simulink library "commrflib2"  (Simulink 6.0)
settings: Solver=ode45  SolverMode=SingleTasking  StartTime=0.0  StopTime=10.0  RelTol=1e-3
undefined symbols (not defined in the file or in its folder): Rows
libraries: dspsigattribs x12, dspmathops x2, commchan2 x2, dsparch3 x1, dspsrcs4 x1
settings Model: Creator=mikem  LastModifiedBy=mikem  ProdHWDeviceType=Microprocessor  TargetHWChar=2  TargetHWWordLengths=8,16,32,32
settings DataIOCC: SignalLoggingName=logsOut
settings OptimizationCC: BooleanDataType=off  MultiInstanced=off
settings FormatCC: IgnoreBidirectionalLines=off
settings HardwareCC: ProdHWDeviceType=Microprocessor  ShiftRightIntArith=on  TargetHWCharacteristics=InheritFromRTWHook
settings CodeAppCC: FileBanners=off
settings GRTTargetCC: TargetFcnLib=iso_c_tmw.mat  IsERTTarget=off

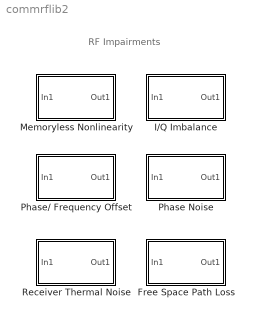
== system commrflib2 ==
  note: RF Impairments
  Free Space Path Loss : Subsystem  mask(Free Space Path Loss){mode=Distance and Frequency, dB=10, d=0.100, fc=1920}
      mask prompts: dB "Loss (dB):"; d "Distance (km):"; fc "Carrier frequency (MHz):"
      mask help:
      | Reduce the amplitude of the input signal by the amount specified.  The loss can be specified directly using the "Decibels" mode, or indirectly using the "Distance and Frequency" mode.
      |
      | The reciprocal of the loss is applied as a gain, e.g., a loss of +20 dB, which reduces the signal by a factor of 10, corresponds to a gain value of 0.1.
      |
      | Note:  The decibel amount shown on the mask is rounded for display purposes only.
      mask init:
      | if mode == 1
      | 
      | 	loss = 10.^(0.05*dB);
      | 
      | else
      | 
      | 	c = 299792458;
      | 
      | 	loss = 4*pi*d*1e3*fc*1e6/c;
      | 
      | end
      | 
      | g = 1/loss;
      | 
      | lossdB = 20*log10(loss);
      | 
      | 
      | 
      | if isempty(dB) | (sum(size(dB)) > 2),
      | 
      | 	dB = 0; g = 0;
      | 
      | 	s = ['Free Space\nPath Loss'];
      | 
      | else
      | 
      | 	s = sprintf('Free Space\nPath Loss\n%0.0f dB',lossdB);
      | 
      | end
      mask Help: helpview(commbhelp)
      mask StyleString: popup(Decibels|Distance and Frequency),edit,edit,edit
      mask CallbackString:
      | if strcmp(get_param(gcb,'mode'),'Decibels'),
      | 
      | 	set_param(gcb,'maskvisibilities',{'on' 'on' 'off' 'off'});
      | 
      | else
      | 
      | 	set_param(gcb,'maskvisibilities',{'on' 'off' 'on' 'on'});
      | 
      | end|||
      mask Display: fprintf(s)
  I/Q Imbalance : Subsystem  mask(I/Q Imbalance){ampImbal=0, phsImbal=0, Idc=0, Qdc=0}
      mask prompts: ampImbal "I/Q amplitude imbalance (dB):"; phsImbal "I/Q phase imbalance (deg):"; Idc "I dc offset:"; Qdc "Q dc offset:"
      mask help: Complex baseband model of the signal impairments caused by imbalances between in-phase and quadrature receiver components.
      mask init:
      | Igain = 10.^(0.5*[ampImbal]*.05);
      | Qgain = 10.^(0.5*[-ampImbal]*.05);
      mask Help: helpview(commbhelp)
      mask Display: disp('I/Q\nImbalance');
  Memoryless Nonlinearity : Subsystem  mask(Memoryless Nonlinearity){model_select=Cubic polynomial, linGaindB=0, GindB=0, iip3=30, am2pm=0, amam=[2.1587 1.1517], ampm=[4.0033 9.1040], x=[8.1081 1.5413 6.5202 -0.0718], y=[4.6645 2.0965 10.88 -0.003], p=0.5, GoutdB=0, vsat=1}
      mask prompts: model_select "Method:"; linGaindB "Linear gain (dB):"; GindB "Input scaling (dB):"; iip3 "IIP3 (dBm):"; am2pm "AM/PM conversion (degrees per dB):"; amam "AM/AM parameters [alpha beta]:"; ampm "AM/PM parameters [alpha beta]:"; x "AM/AM parameters [x1 x2 x3 x4]:"; y "AM/PM parameters [y1 y2 y3 y4]:"; p "Smoothness factor:"; GoutdB "Output scaling (dB):"; vsat "Output saturation level:"
      mask help:
      | Complex baseband model of memoryless nonlinearity.
      |
      | Two of the five methods (Cubic Polynomial and Hyperbolic Tangent) fit curves to measured data provided by the gain and third order intercept point (IIP3) parameters.
      |
      | The other three methods use models originated by Saleh, Ghorbani, and Rapp.  The Saleh and Ghorbani models are based on normalized nonlinear transfer functions.  Use the Input scaling and Output scaling parameters to adjust signal levels up or down from their normalized values.
      mask init:
      | switch model_select
      | case 'Cubic polynomial'
      |     str = ['Cubic\nPolynomial'];
      |     method = 1;
      | 	c1 = 10^(linGaindB/20);
      |     inputGain = sqrt(3/(10^((iip3-30)/10)));
      |     outputGain = c1/inputGain;
      | case 'Hyperbolic tangent'
      |     str = ['Hyperbolic\nTangent'];
      |     method = 2;
      | 	c1 = 10^(linGaindB/20);
      |     inputGain = sqrt(3/(10^((iip3-30)/10)));
      |     outputGain = c1/inputGain;
      | case 'Saleh model',
      |     str = ['Saleh\nModel'];
      |     method = 3;
      |     inputGain = 10^(GindB/20);
      |     outputGain = 10^(GoutdB/20);
      | case 'Ghorbani model',
      |     str = ['Ghorbani\nModel'];
      |     method = 4;
      |     inputGain = 10^(GindB/20);
      |     outputGain = 10^(GoutdB/20);
      | case 'Rapp model',
      |     str = ['Rapp\nModel'];
      |     method = 5;
      | 	c1 = 10^(linGaindB/20);
      |     inputGain = c1;
      |     outputGain = 1;
      | end
      mask Help: helpview(commbhelp)
      mask StyleString: popup(Cubic polynomial|Hyperbolic tangent|Saleh model|Ghorbani model|Rapp model),edit,edit,edit,edit,edit,edit,edit,edit,edit,edit,edit
      mask CallbackString:
      | model_type = get_param(gcb,'model_select');
      | 
      | switch model_type
      | 
      | case 'Cubic polynomial',
      | 
      | 	set_param(gcb,'maskvisibilities',{'on' 'on' 'off' 'on' 'on' 'off' 'off' 'off' 'off' 'off' 'off' 'off'});
      | 
      | case 'Hyperbolic tangent',
      | 
      | 	set_param(gcb,'maskvisibilities',{'on' 'on' 'off' 'on' 'on' 'off' 'off' 'off' 'off' 'off' 'off' 'off'});
      | 
      | case 'Saleh model',
      | 
      | 	set_param(gcb,'maskvisibilities',{'on' 'off' 'on' 'off' 'off' 'on' 'on' 'off' 'off' 'off' 'on' 'off'});
      | 
      | case 'Ghorbani model',
      | 
      | 	set_param(gcb,'maskvisibilities',{'on' 'off' 'on' 'off' 'off' 'off' 'off' 'on' 'on' 'off' 'on' 'off'});
      | 
      | case 'Rapp model',
      | 
      | 	set_param(gcb,'maskvisibilities',{'on' 'on' 'off' 'off' 'off' 'off' 'off' 'off' 'off' 'on' 'off' 'on'});
      | 
      | end|||||||||||
      mask Display: disp(str);
  Phase Noise : Subsystem  mask(Phase Noise){PhNs=-120, Fo=100, seed=2137}
      mask prompts: PhNs "Phase noise level (dBc/Hz):"; Fo "Frequency offset (Hz):"; seed "Initial seed:"
      mask help:
      | Complex baseband model of receiver phase noise.
      |
      | The output of this block is noise with a spectrum characterized by a 1/f slope.  The level of the spectrum is specified by the noise power contained in a one hertz bandwidth offset from the carrier by a certain frequency.
      mask init:
      | if PhNs>0,
      | 	error('Phase noise level should be negative.');
      | end
      | num = sqrt(2*pi*Fo*10^((PhNs)/10));
      | if num>.1,
      | 	warning('Current parameters in phase noise block may produce inaccurate results.');
      | end
      | num_taps = 64;
      | den = zeros(1,num_taps);
      | den(1) = 1;
      | for idx = 2:num_taps
      |    den(idx) = (idx - 2.5) * den(idx-1) / (idx-1);
      | end
      settings: AttributesFormatString=\n
      mask Help: helpview(commbhelp)
      mask Display: disp('Phase\nNoise');
  Phase/ Frequency Offset : Subsystem  mask(Phase/Frequency Offset){freqOffset=0, phaseOffset=0}
      mask prompts: freqOffset "Frequency offset (Hz):"; phaseOffset "Phase offset (deg):"
      mask help: Complex baseband model of residual phase and frequency offsets.
      mask Help: helpview(commbhelp)
      mask Display: disp('Phase/\nFrequency\nOffset');
  Receiver Thermal Noise : Subsystem  mask(Receiver Thermal Noise){method=Noise temperature, ntemp=290, nfigure=3.01, nfactor=2, seed=67987}
      mask prompts: method "Specification method:"; ntemp "Noise temperature (K):"; nfigure "Noise figure (dB):"; nfactor "Noise factor:"; seed "Initial seed:"
      mask help:
      | Complex baseband model of receiver thermal noise.
      |
      | The amount of noise added to the input signal may be specified either in terms of noise temperature, noise figure, or noise factor.
      mask init:
      | k=1.380650e-23; % Boltzmann's constant, J/K
      | 
      | switch method
      | case 'Noise temperature',
      | 	T = ntemp;
      | 	str = ['Noise\nTemperature\n' num2str(ntemp) ' K'];
      | case 'Noise figure',
      | 	nfactor = 10.^(0.1*nfigure);
      | 	T = 290*(nfactor-1);
      | 	str = ['Noise\nFigure\n' num2str(nfigure) ' dB'];
      | case 'Noise factor',
      | 	T = 290*(nfactor-1);
      | 	str = ['Noise\nFactor\n' num2str(nfactor)];
      | end
      | 
      | kT=k*T;
      mask Help: helpview(commbhelp)
      mask StyleString: popup(Noise temperature|Noise figure|Noise factor),edit,edit,edit,edit
      mask CallbackString:
      | method = get_param(gcb,'method');
      | 
      | switch method
      | 
      | case 'Noise temperature',
      | 
      | 	set_param(gcb,'maskvisibilities',{'on' 'on' 'off' 'off' 'on'});
      | 
      | case 'Noise figure',
      | 
      | 	set_param(gcb,'maskvisibilities',{'on' 'off' 'on' 'off' 'on'});
      | 
      | case 'Noise factor',
      | 
      | 	set_param(gcb,'maskvisibilities',{'on' 'off' 'off' 'on' 'on'});
      | 
      | end||||
      mask Display: disp(str);

== system commrflib2/Free Space Path Loss ==
  In1 : Inport
  Check Input Signal : Subsystem
      mask Display: disp('Check\nInput Signal');
  Gain : Gain  Gain=g  SaturateOnIntegerOverflow=on
  Out1 : Outport
  wires:
  In1/1 -> Check Input Signal/1(In1)
  Gain/1 -> Out1/1
  Check Input Signal/1(Out1) -> Gain/1

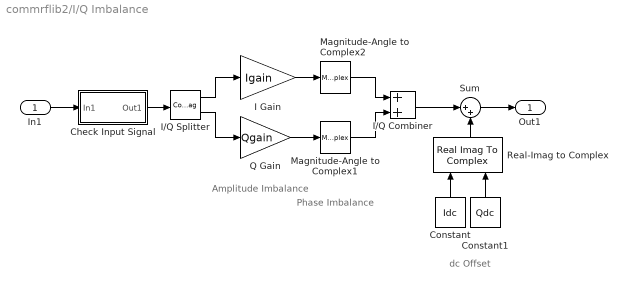
== system commrflib2/I/Q Imbalance ==
  note: Amplitude
      | Imbalance
  note: Phase
      | Imbalance
  note: dc
      | Offset
  In1 : Inport
  Check Input Signal : Subsystem
      mask Display: disp('Check\nInput Signal');
  Constant : Constant  Orientation=up  Value=Idc
  Constant1 : Constant  Orientation=up  Value=Qdc
  I Gain : Gain  Gain=Igain  SaturateOnIntegerOverflow=on
  I/Q Combiner : Sum  SaturateOnIntegerOverflow=on  InputSameDT=on
  I/Q Splitter : ComplexToRealImag
  Magnitude-Angle to Complex1 : MagnitudeAngleToComplex  Input=Magnitude  ConstantPart=pi/2+0.5*phsImbal*pi/180
  Magnitude-Angle to Complex2 : MagnitudeAngleToComplex  Input=Magnitude  ConstantPart=-0.5*phsImbal*pi/180
  Q Gain : Gain  Gain=Qgain  SaturateOnIntegerOverflow=on
  Real-Imag to Complex : RealImagToComplex  Orientation=up
  Sum : Sum  Inputs=|++  SaturateOnIntegerOverflow=on  InputSameDT=on
  Out1 : Outport
  wires:
  I/Q Splitter/1 -> I Gain/1
  I/Q Splitter/2 -> Q Gain/1
  I Gain/1 -> Magnitude-Angle to Complex2/1
  Q Gain/1 -> Magnitude-Angle to Complex1/1
  In1/1 -> Check Input Signal/1(In1)
  Sum/1 -> Out1/1
  Check Input Signal/1(Out1) -> I/Q Splitter/1
  Magnitude-Angle to Complex2/1 -> I/Q Combiner/1
  Magnitude-Angle to Complex1/1 -> I/Q Combiner/2
  I/Q Combiner/1 -> Sum/1
  Constant/1 -> Real-Imag to Complex/1
  Constant1/1 -> Real-Imag to Complex/2
  Real-Imag to Complex/1 -> Sum/2

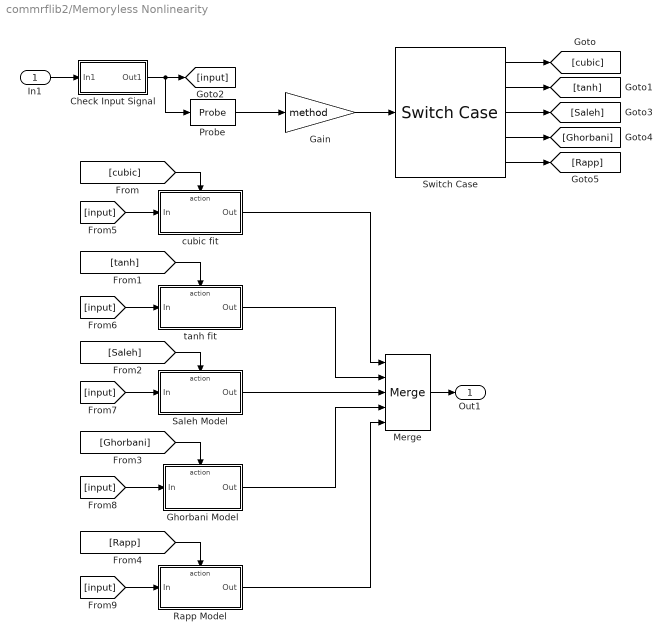
== system commrflib2/Memoryless Nonlinearity ==
  In1 : Inport
  Check Input Signal : Subsystem
      mask Display: disp('Check\nInput Signal');
  Gain : Gain  Gain=method  SaturateOnIntegerOverflow=on
  Ghorbani Model : Subsystem  TreatAsAtomicUnit=on
  Merge : Merge  Inputs=5
  Probe : Probe  ProbeWidth=off  ProbeSampleTime=off
  Rapp Model : Subsystem  TreatAsAtomicUnit=on
  Saleh Model : Subsystem  TreatAsAtomicUnit=on
  Switch Case : SwitchCase  CaseConditions={1 2 3 4 5}  CaseShowDefault=off
  cubic fit : Subsystem  TreatAsAtomicUnit=on
  tanh fit : Subsystem  TreatAsAtomicUnit=on
  Out1 : Outport
  wires:
  Gain/1 -> Switch Case/1
  Merge/1 -> Out1/1
  tanh fit/1(Out) -> Merge/2
  cubic fit/1(Out) -> Merge/1
  [cubic] -> cubic fit/Action
  [tanh] -> tanh fit/Action
  Switch Case/2 -> [tanh]
  In1/1 -> Check Input Signal/1(In1)
  Check Input Signal/1(Out1) -> [input], Probe/1
  [Rapp] -> Rapp Model/Action
  [Ghorbani] -> Ghorbani Model/Action
  [Saleh] -> Saleh Model/Action
  Switch Case/3 -> [Saleh]
  Switch Case/4 -> [Ghorbani]
  Switch Case/5 -> [Rapp]
  Saleh Model/1(Out) -> Merge/3
  Rapp Model/1(Out) -> Merge/5
  [input] -> cubic fit/1(In)
  [input] -> Rapp Model/1(In)
  [input] -> Ghorbani Model/1(In)
  [input] -> Saleh Model/1(In)
  [input] -> tanh fit/1(In)
  Ghorbani Model/1(Out) -> Merge/4
  Switch Case/1 -> [cubic]
  Probe/1 -> Gain/1

== system commrflib2/Phase Noise ==
  In1 : Inport
  Check Input Signal : Subsystem
      mask Display: disp('Check\nInput Signal');
  Digital Filter : dsparch3/Direct-Form II Transpose Filter  num=num  den=den  ic=0
  Magnitude-Angle to Complex : MagnitudeAngleToComplex  Input=Angle  ConstantPart=1
  Noise Source : Subsystem
      mask Display: disp('Noise Source')
  Product : Product  SaturateOnIntegerOverflow=on  InputSameDT=on
  Out1 : Outport
  wires:
  Noise Source/1(Out1) -> Digital Filter/1
  Product/1 -> Out1/1
  In1/1 -> Check Input Signal/1(In1)
  Magnitude-Angle to Complex/1 -> Product/2
  Digital Filter/1 -> Magnitude-Angle to Complex/1
  Check Input Signal/1(Out1) -> Product/1, Noise Source/1(In1)

== system commrflib2/Phase/ Frequency Offset ==
  In1 : Inport
  Check Input Signal : Subsystem
      mask Display: disp('Check\nInput Signal');
  Frequency Offset : Subsystem
      mask Display: disp('Frequency\nOffset');
  Phase Offset : Subsystem
      mask Display: disp('Phase\nOffset');
  Out1 : Outport
  wires:
  Frequency Offset/1(Out1) -> Out1/1
  In1/1 -> Check Input Signal/1(In1)
  Phase Offset/1(Out1) -> Frequency Offset/1(In1)
  Check Input Signal/1(Out1) -> Phase Offset/1(In1)

== system commrflib2/Receiver Thermal Noise ==
  In1 : Inport
  AWGN Noise Temp : commchan2/AWGN Channel  seed=seed  noiseMode=Variance from port  EbNodB=10  EsNodB=10  SNRdB=10  bitsPerSym=1  Ps=1  Tsym=1  variance=var
  Check Input Signal : Subsystem
      mask Display: disp('Check\nInput Signal');
  Gain : Gain  Gain=kT  SaturateOnIntegerOverflow=on
  Probe : Probe  ProbeComplexSignal=off
  Product : Product  Inputs=*/  SaturateOnIntegerOverflow=on  InputSameDT=on
  Selector : Selector  InputPortWidth=2
  Out1 : Outport
  wires:
  AWGN Noise Temp/1 -> Out1/1
  In1/1 -> Check Input Signal/1(In1)
  Probe/1 -> Product/1
  Product/1 -> Gain/1
  Gain/1 -> AWGN Noise Temp/2
  Probe/2 -> Selector/1
  Selector/1 -> Product/2
  Check Input Signal/1(Out1) -> AWGN Noise Temp/1, Probe/1

== system commrflib2/Free Space Path Loss/Check Input Signal ==
  In1 : Inport
  Check Signal Attributes : dspsigattribs/Check Signal Attributes  SigAttribCheckMethod=Does not match attributes exactly  Complexity=Complex  Frame=Ignore  DimsCheckMethod=Is...  Dimensions=Column vector (2-D) or scalar  DatatypeCheckMethod=Ignore  DatatypeGeneral=Boolean  DtypeFloatSpecific=Any floating-point  DtypeFixedSpecific=Any fixed-point  DtypeIntSpecific=Any integer  SampleMode=Ignore
  Check Signal Attributes1 : dspsigattribs/Check Signal Attributes  SigAttribCheckMethod=Matches attributes exactly  Complexity=Ignore  Frame=Sample-based  DimsCheckMethod=Is...  Dimensions=Vector (1-D or 2-D)  DatatypeCheckMethod=Ignore  DatatypeGeneral=Boolean  DtypeFloatSpecific=Any floating-point  DtypeFixedSpecific=Any fixed-point  DtypeIntSpecific=Any integer  SampleMode=Ignore
  Out1 : Outport
  wires:
  In1/1 -> Check Signal Attributes/1
  Check Signal Attributes1/1 -> Out1/1
  Check Signal Attributes/1 -> Check Signal Attributes1/1

== system commrflib2/I/Q Imbalance/Check Input Signal ==
  In1 : Inport
  Check Signal Attributes : dspsigattribs/Check Signal Attributes  SigAttribCheckMethod=Does not match attributes exactly  Complexity=Complex  Frame=Ignore  DimsCheckMethod=Is...  Dimensions=Column vector (2-D) or scalar  DatatypeCheckMethod=Ignore  DatatypeGeneral=Boolean  DtypeFloatSpecific=Any floating-point  DtypeFixedSpecific=Any fixed-point  DtypeIntSpecific=Any integer  SampleMode=Ignore
  Check Signal Attributes1 : dspsigattribs/Check Signal Attributes  SigAttribCheckMethod=Matches attributes exactly  Complexity=Ignore  Frame=Sample-based  DimsCheckMethod=Is...  Dimensions=Vector (1-D or 2-D)  DatatypeCheckMethod=Ignore  DatatypeGeneral=Boolean  DtypeFloatSpecific=Any floating-point  DtypeFixedSpecific=Any fixed-point  DtypeIntSpecific=Any integer  SampleMode=Ignore
  Out1 : Outport
  wires:
  Check Signal Attributes/1 -> Check Signal Attributes1/1
  Check Signal Attributes1/1 -> Out1/1
  In1/1 -> Check Signal Attributes/1

== system commrflib2/Memoryless Nonlinearity/Check Input Signal ==
  In1 : Inport
  Check Signal Attributes : dspsigattribs/Check Signal Attributes  SigAttribCheckMethod=Does not match attributes exactly  Complexity=Complex  Frame=Ignore  DimsCheckMethod=Is...  Dimensions=Column vector (2-D) or scalar  DatatypeCheckMethod=Ignore  DatatypeGeneral=Boolean  DtypeFloatSpecific=Any floating-point  DtypeFixedSpecific=Any fixed-point  DtypeIntSpecific=Any integer  SampleMode=Ignore
  Check Signal Attributes1 : dspsigattribs/Check Signal Attributes  SigAttribCheckMethod=Matches attributes exactly  Complexity=Ignore  Frame=Sample-based  DimsCheckMethod=Is...  Dimensions=Vector (1-D or 2-D)  DatatypeCheckMethod=Ignore  DatatypeGeneral=Boolean  DtypeFloatSpecific=Any floating-point  DtypeFixedSpecific=Any fixed-point  DtypeIntSpecific=Any integer  SampleMode=Ignore
  Out1 : Outport
  wires:
  In1/1 -> Check Signal Attributes/1
  Check Signal Attributes1/1 -> Out1/1
  Check Signal Attributes/1 -> Check Signal Attributes1/1

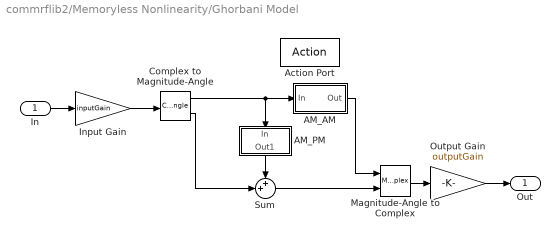
== system commrflib2/Memoryless Nonlinearity/Ghorbani Model ==
  In : Inport
  Action Port : ActionPort
  AM_AM : Subsystem
      mask Display: disp('AM/AM')
  AM_PM : Subsystem  Orientation=down
      mask Display: disp('AM/PM')
  Complex to Magnitude-Angle : ComplexToMagnitudeAngle
  Input Gain : Gain  Gain=inputGain  SaturateOnIntegerOverflow=on
  Magnitude-Angle to Complex : MagnitudeAngleToComplex
  Output Gain : Gain  Gain=outputGain  SaturateOnIntegerOverflow=on
  Sum : Sum  Inputs=++|  SaturateOnIntegerOverflow=on  InputSameDT=on
  Out : Outport
  wires:
  Sum/1 -> Magnitude-Angle to Complex/2
  AM_PM/1(Out1) -> Sum/1
  Output Gain/1 -> Out/1
  In/1 -> Input Gain/1
  Complex to Magnitude-Angle/2 -> Sum/2
  Input Gain/1 -> Complex to Magnitude-Angle/1
  Magnitude-Angle to Complex/1 -> Output Gain/1
  AM_AM/1(Out) -> Magnitude-Angle to Complex/1
  Complex to Magnitude-Angle/1 -> AM_AM/1(In), AM_PM/1(In)

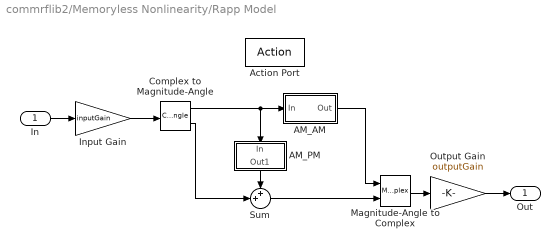
== system commrflib2/Memoryless Nonlinearity/Rapp Model ==
  In : Inport
  Action Port : ActionPort
  AM_AM : Subsystem
      mask Display: disp('AM/AM')
  AM_PM : Subsystem  Orientation=down
      mask Display: disp('AM/PM')
  Complex to Magnitude-Angle : ComplexToMagnitudeAngle
  Input Gain : Gain  Gain=inputGain  SaturateOnIntegerOverflow=on
  Magnitude-Angle to Complex : MagnitudeAngleToComplex
  Output Gain : Gain  Gain=outputGain  SaturateOnIntegerOverflow=on
  Sum : Sum  Inputs=++|  SaturateOnIntegerOverflow=on  InputSameDT=on
  Out : Outport
  wires:
  Output Gain/1 -> Out/1
  In/1 -> Input Gain/1
  Input Gain/1 -> Complex to Magnitude-Angle/1
  Magnitude-Angle to Complex/1 -> Output Gain/1
  AM_AM/1(Out) -> Magnitude-Angle to Complex/1
  Complex to Magnitude-Angle/1 -> AM_AM/1(In), AM_PM/1(In)
  AM_PM/1(Out1) -> Sum/1
  Complex to Magnitude-Angle/2 -> Sum/2
  Sum/1 -> Magnitude-Angle to Complex/2

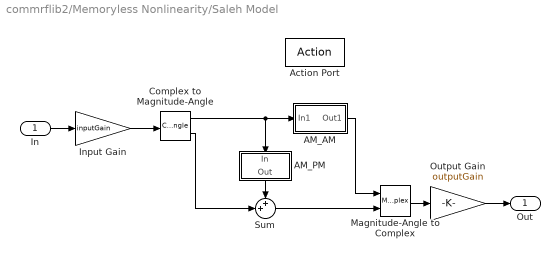
== system commrflib2/Memoryless Nonlinearity/Saleh Model ==
  In : Inport
  Action Port : ActionPort
  AM_AM : Subsystem
      mask Display: disp('AM/AM')
  AM_PM : Subsystem  Orientation=down
      mask Display: disp('AM/PM')
  Complex to Magnitude-Angle : ComplexToMagnitudeAngle
  Input Gain : Gain  Gain=inputGain  SaturateOnIntegerOverflow=on
  Magnitude-Angle to Complex : MagnitudeAngleToComplex
  Output Gain : Gain  Gain=outputGain  SaturateOnIntegerOverflow=on
  Sum : Sum  Inputs=++|  SaturateOnIntegerOverflow=on  InputSameDT=on
  Out : Outport
  wires:
  Sum/1 -> Magnitude-Angle to Complex/2
  AM_PM/1(Out) -> Sum/1
  Output Gain/1 -> Out/1
  In/1 -> Input Gain/1
  Complex to Magnitude-Angle/2 -> Sum/2
  Input Gain/1 -> Complex to Magnitude-Angle/1
  Magnitude-Angle to Complex/1 -> Output Gain/1
  AM_AM/1(Out1) -> Magnitude-Angle to Complex/1
  Complex to Magnitude-Angle/1 -> AM_AM/1(In1), AM_PM/1(In)

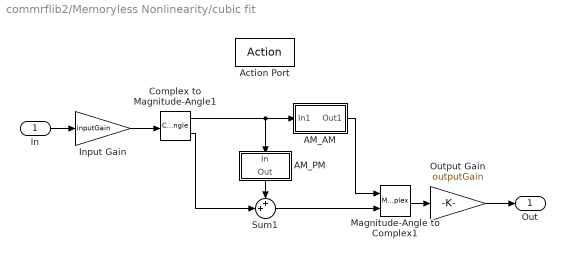
== system commrflib2/Memoryless Nonlinearity/cubic fit ==
  In : Inport
  Action Port : ActionPort
  AM_AM : Subsystem
      mask Display: disp('AM/AM')
  AM_PM : Subsystem  Orientation=down
      mask Display: disp('AM/PM')
  Complex to Magnitude-Angle1 : ComplexToMagnitudeAngle
  Input Gain : Gain  Gain=inputGain  SaturateOnIntegerOverflow=on
  Magnitude-Angle to Complex1 : MagnitudeAngleToComplex
  Output Gain : Gain  Gain=outputGain  SaturateOnIntegerOverflow=on
  Sum1 : Sum  Inputs=++|  SaturateOnIntegerOverflow=on  InputSameDT=on
  Out : Outport
  wires:
  Complex to Magnitude-Angle1/1 -> AM_AM/1(In1), AM_PM/1(In)
  AM_AM/1(Out1) -> Magnitude-Angle to Complex1/1
  Magnitude-Angle to Complex1/1 -> Output Gain/1
  Input Gain/1 -> Complex to Magnitude-Angle1/1
  Complex to Magnitude-Angle1/2 -> Sum1/2
  In/1 -> Input Gain/1
  Output Gain/1 -> Out/1
  AM_PM/1(Out) -> Sum1/1
  Sum1/1 -> Magnitude-Angle to Complex1/2

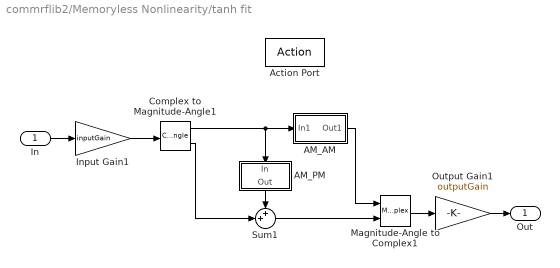
== system commrflib2/Memoryless Nonlinearity/tanh fit ==
  In : Inport
  Action Port : ActionPort
  AM_AM : Subsystem
      mask Display: disp('AM/AM')
  AM_PM : Subsystem  Orientation=down
      mask Display: disp('AM/PM')
  Complex to Magnitude-Angle1 : ComplexToMagnitudeAngle
  Input Gain1 : Gain  Gain=inputGain  SaturateOnIntegerOverflow=on
  Magnitude-Angle to Complex1 : MagnitudeAngleToComplex
  Output Gain1 : Gain  Gain=outputGain  SaturateOnIntegerOverflow=on
  Sum1 : Sum  Inputs=++|  SaturateOnIntegerOverflow=on  InputSameDT=on
  Out : Outport
  wires:
  Complex to Magnitude-Angle1/1 -> AM_AM/1(In1), AM_PM/1(In)
  AM_AM/1(Out1) -> Magnitude-Angle to Complex1/1
  Magnitude-Angle to Complex1/1 -> Output Gain1/1
  Input Gain1/1 -> Complex to Magnitude-Angle1/1
  Complex to Magnitude-Angle1/2 -> Sum1/2
  In/1 -> Input Gain1/1
  Output Gain1/1 -> Out/1
  AM_PM/1(Out) -> Sum1/1
  Sum1/1 -> Magnitude-Angle to Complex1/2

== system commrflib2/Phase Noise/Check Input Signal ==
  In1 : Inport
  Check Signal Attributes : dspsigattribs/Check Signal Attributes  SigAttribCheckMethod=Does not match attributes exactly  Complexity=Complex  Frame=Ignore  DimsCheckMethod=Is...  Dimensions=Column vector (2-D) or scalar  DatatypeCheckMethod=Ignore  DatatypeGeneral=Boolean  DtypeFloatSpecific=Any floating-point  DtypeFixedSpecific=Any fixed-point  DtypeIntSpecific=Any integer  SampleMode=Ignore
  Check Signal Attributes1 : dspsigattribs/Check Signal Attributes  SigAttribCheckMethod=Matches attributes exactly  Complexity=Ignore  Frame=Sample-based  DimsCheckMethod=Is...  Dimensions=Vector (1-D or 2-D)  DatatypeCheckMethod=Ignore  DatatypeGeneral=Boolean  DtypeFloatSpecific=Any floating-point  DtypeFixedSpecific=Any fixed-point  DtypeIntSpecific=Any integer  SampleMode=Ignore
  Out1 : Outport
  wires:
  Check Signal Attributes/1 -> Check Signal Attributes1/1
  Check Signal Attributes1/1 -> Out1/1
  In1/1 -> Check Signal Attributes/1

== system commrflib2/Phase Noise/Noise Source ==
  In1 : Inport  Orientation=down
  AWGN Channel : commchan2/AWGN Channel  seed=seed  noiseMode=Variance from mask  EsNodB=10  SNRdB=0  Ps=1  Tsym=1  variance=2
  Complex to Real-Imag : ComplexToRealImag  Output=Real
  Sum : Sum  Inputs=-+|  SaturateOnIntegerOverflow=on  InputSameDT=on
  Out1 : Outport
  wires:
  Sum/1 -> Complex to Real-Imag/1
  AWGN Channel/1 -> Sum/2
  In1/1 -> AWGN Channel/1, Sum/1
  Complex to Real-Imag/1 -> Out1/1

== system commrflib2/Phase/ Frequency Offset/Check Input Signal ==
  In1 : Inport
  Check Signal Attributes : dspsigattribs/Check Signal Attributes  SigAttribCheckMethod=Does not match attributes exactly  Complexity=Complex  Frame=Ignore  DimsCheckMethod=Is...  Dimensions=Column vector (2-D) or scalar  DatatypeCheckMethod=Ignore  DatatypeGeneral=Boolean  DtypeFloatSpecific=Any floating-point  DtypeFixedSpecific=Any fixed-point  DtypeIntSpecific=Any integer  SampleMode=Ignore
  Check Signal Attributes1 : dspsigattribs/Check Signal Attributes  SigAttribCheckMethod=Matches attributes exactly  Complexity=Ignore  Frame=Sample-based  DimsCheckMethod=Is...  Dimensions=Vector (1-D or 2-D)  DatatypeCheckMethod=Ignore  DatatypeGeneral=Boolean  DtypeFloatSpecific=Any floating-point  DtypeFixedSpecific=Any fixed-point  DtypeIntSpecific=Any integer  SampleMode=Ignore
  Out1 : Outport
  wires:
  Check Signal Attributes/1 -> Check Signal Attributes1/1
  Check Signal Attributes1/1 -> Out1/1
  In1/1 -> Check Signal Attributes/1

== system commrflib2/Phase/ Frequency Offset/Frequency Offset ==
  In1 : Inport
  Calculate Frequency Offset : Subsystem
      mask Display: disp('Calculate\nFrequency\nOffset');
  Product : Product  SaturateOnIntegerOverflow=on  InputSameDT=on
  Out1 : Outport
  wires:
  Product/1 -> Out1/1
  In1/1 -> Product/1, Calculate Frequency Offset/1(In1)
  Calculate Frequency Offset/1(Out1) -> Product/2

== system commrflib2/Phase/ Frequency Offset/Phase Offset ==
  In1 : Inport
  Complex to Magnitude-Angle : ComplexToMagnitudeAngle
  Magnitude-Angle to Complex1 : MagnitudeAngleToComplex  Input=Angle  ConstantPart=1
  Magnitude-Angle to Complex2 : MagnitudeAngleToComplex  Input=Magnitude  ConstantPart=phaseOffset*pi/180
  Product : Product  SaturateOnIntegerOverflow=on  InputSameDT=on
  Out1 : Outport
  wires:
  Complex to Magnitude-Angle/2 -> Magnitude-Angle to Complex1/1
  Complex to Magnitude-Angle/1 -> Magnitude-Angle to Complex2/1
  Magnitude-Angle to Complex2/1 -> Product/1
  Magnitude-Angle to Complex1/1 -> Product/2
  In1/1 -> Complex to Magnitude-Angle/1
  Product/1 -> Out1/1

== system commrflib2/Receiver Thermal Noise/Check Input Signal ==
  In1 : Inport
  Check Signal Attributes : dspsigattribs/Check Signal Attributes  SigAttribCheckMethod=Does not match attributes exactly  Complexity=Complex  Frame=Ignore  DimsCheckMethod=Is...  Dimensions=Column vector (2-D) or scalar  DatatypeCheckMethod=Ignore  DatatypeGeneral=Boolean  DtypeFloatSpecific=Any floating-point  DtypeFixedSpecific=Any fixed-point  DtypeIntSpecific=Any integer  SampleMode=Ignore
  Check Signal Attributes1 : dspsigattribs/Check Signal Attributes  SigAttribCheckMethod=Matches attributes exactly  Complexity=Ignore  Frame=Sample-based  DimsCheckMethod=Is...  Dimensions=Vector (1-D or 2-D)  DatatypeCheckMethod=Ignore  DatatypeGeneral=Boolean  DtypeFloatSpecific=Any floating-point  DtypeFixedSpecific=Any fixed-point  DtypeIntSpecific=Any integer  SampleMode=Ignore
  Out1 : Outport
  wires:
  In1/1 -> Check Signal Attributes/1
  Check Signal Attributes1/1 -> Out1/1
  Check Signal Attributes/1 -> Check Signal Attributes1/1

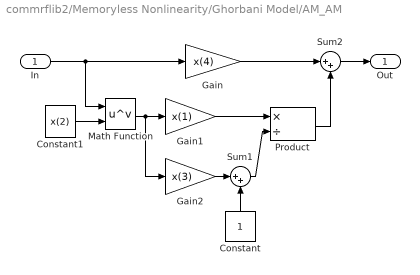
== system commrflib2/Memoryless Nonlinearity/Ghorbani Model/AM_AM ==
  In : Inport
  Constant : Constant  Orientation=up
  Constant1 : Constant  Value=x(2)
  Gain : Gain  Gain=x(4)  SaturateOnIntegerOverflow=on
  Gain1 : Gain  Gain=x(1)  SaturateOnIntegerOverflow=on
  Gain2 : Gain  Gain=x(3)  SaturateOnIntegerOverflow=on
  Math Function : Math  Operator=pow
  Product : Product  Inputs=*/  SaturateOnIntegerOverflow=on  InputSameDT=on
  Sum1 : Sum  Inputs=|++  SaturateOnIntegerOverflow=on  InputSameDT=on
  Sum2 : Sum  Inputs=|++  SaturateOnIntegerOverflow=on  InputSameDT=on
  Out : Outport
  wires:
  Sum2/1 -> Out/1
  In/1 -> Math Function/1, Gain/1
  Sum1/1 -> Product/2
  Gain2/1 -> Sum1/1
  Constant/1 -> Sum1/2
  Product/1 -> Sum2/2
  Gain1/1 -> Product/1
  Constant1/1 -> Math Function/2
  Math Function/1 -> Gain2/1, Gain1/1
  Gain/1 -> Sum2/1

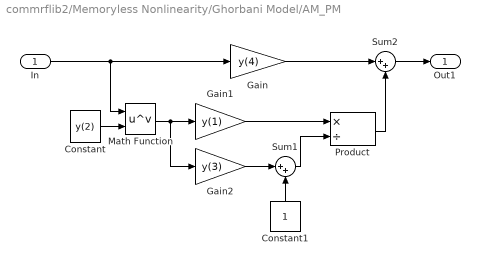
== system commrflib2/Memoryless Nonlinearity/Ghorbani Model/AM_PM ==
  In : Inport
  Constant : Constant  Value=y(2)
  Constant1 : Constant  Orientation=up
  Gain : Gain  Gain=y(4)  SaturateOnIntegerOverflow=on
  Gain1 : Gain  Gain=y(1)  SaturateOnIntegerOverflow=on
  Gain2 : Gain  Gain=y(3)  SaturateOnIntegerOverflow=on
  Math Function : Math  Operator=pow
  Product : Product  Inputs=*/  SaturateOnIntegerOverflow=on  InputSameDT=on
  Sum1 : Sum  Inputs=|++  SaturateOnIntegerOverflow=on  InputSameDT=on
  Sum2 : Sum  Inputs=|++  SaturateOnIntegerOverflow=on  InputSameDT=on
  Out1 : Outport
  wires:
  Sum2/1 -> Out1/1
  In/1 -> Gain/1, Math Function/1
  Sum1/1 -> Product/2
  Gain2/1 -> Sum1/1
  Constant1/1 -> Sum1/2
  Product/1 -> Sum2/2
  Gain1/1 -> Product/1
  Constant/1 -> Math Function/2
  Math Function/1 -> Gain1/1, Gain2/1
  Gain/1 -> Sum2/1

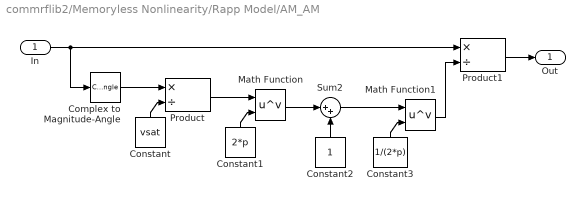
== system commrflib2/Memoryless Nonlinearity/Rapp Model/AM_AM ==
  In : Inport
  Complex to Magnitude-Angle : ComplexToMagnitudeAngle  Output=Magnitude
  Constant : Constant  Orientation=up  Value=vsat
  Constant1 : Constant  Orientation=up  Value=2*p
  Constant2 : Constant  Orientation=up
  Constant3 : Constant  Orientation=up  Value=1/(2*p)
  Math Function : Math  Operator=pow
  Math Function1 : Math  Operator=pow
  Product : Product  Inputs=*/  SaturateOnIntegerOverflow=on  InputSameDT=on
  Product1 : Product  Inputs=*/  SaturateOnIntegerOverflow=on  InputSameDT=on
  Sum2 : Sum  Inputs=|++  SaturateOnIntegerOverflow=on  InputSameDT=on
  Out : Outport
  wires:
  Product1/1 -> Out/1
  In/1 -> Product1/1, Complex to Magnitude-Angle/1
  Constant/1 -> Product/2
  Constant2/1 -> Sum2/2
  Product/1 -> Math Function/1
  Math Function/1 -> Sum2/1
  Constant1/1 -> Math Function/2
  Complex to Magnitude-Angle/1 -> Product/1
  Sum2/1 -> Math Function1/1
  Constant3/1 -> Math Function1/2
  Math Function1/1 -> Product1/2

== system commrflib2/Memoryless Nonlinearity/Rapp Model/AM_PM ==
  In : Inport
  Ground : Ground
  Terminator : Terminator
  Out1 : Outport
  wires:
  In/1 -> Terminator/1
  Ground/1 -> Out1/1

== system commrflib2/Memoryless Nonlinearity/Saleh Model/AM_AM ==
  In1 : Inport
  Constant1 : Constant
  Gain2 : Gain  Gain=amam(2)  SaturateOnIntegerOverflow=on
  Gain3 : Gain  Gain=amam(1)  SaturateOnIntegerOverflow=on
  Math Function : Math  Operator=square
  Product2 : Product  Inputs=*/  SaturateOnIntegerOverflow=on  InputSameDT=on
  Sum1 : Sum  Inputs=|++  SaturateOnIntegerOverflow=on  InputSameDT=on
  Out1 : Outport
  wires:
  Product2/1 -> Out1/1
  In1/1 -> Gain3/1, Math Function/1
  Gain3/1 -> Product2/1
  Sum1/1 -> Product2/2
  Constant1/1 -> Sum1/2
  Gain2/1 -> Sum1/1
  Math Function/1 -> Gain2/1

== system commrflib2/Memoryless Nonlinearity/Saleh Model/AM_PM ==
  In : Inport
  Constant : Constant  Orientation=up
  Gain : Gain  Gain=ampm(2)  SaturateOnIntegerOverflow=on
  Gain1 : Gain  Gain=ampm(1)  SaturateOnIntegerOverflow=on
  Math Function : Math  Operator=square
  Product : Product  Inputs=*/  SaturateOnIntegerOverflow=on  InputSameDT=on
  Sum : Sum  Inputs=|++  SaturateOnIntegerOverflow=on  InputSameDT=on
  Out : Outport
  wires:
  In/1 -> Math Function/1
  Math Function/1 -> Gain/1, Gain1/1
  Product/1 -> Out/1
  Gain/1 -> Sum/1
  Constant/1 -> Sum/2
  Sum/1 -> Product/2
  Gain1/1 -> Product/1

== system commrflib2/Memoryless Nonlinearity/cubic fit/AM_AM ==
  In1 : Inport
  Constant : Constant  Value=3
  Gain : Gain  Gain=1/3  SaturateOnIntegerOverflow=on
  Math Function : Math  Operator=pow
  Saturation I : Saturate  UpperLimit=1  LowerLimit=-1
  Sum : Sum  Inputs=+-|  SaturateOnIntegerOverflow=on  InputSameDT=on
  Out1 : Outport
  wires:
  Sum/1 -> Out1/1
  Saturation I/1 -> Math Function/1, Sum/1
  Math Function/1 -> Gain/1
  Constant/1 -> Math Function/2
  Gain/1 -> Sum/2
  In1/1 -> Saturation I/1

== system commrflib2/Memoryless Nonlinearity/cubic fit/AM_PM ==
  In : Inport
  Input Gain : Gain  Gain=am2pm*pi/180  SaturateOnIntegerOverflow=on
  dB Conversion : dspmathops/dB Conversion  dBtype=dB  intype=Amplitude  R=1  fuzz=on
  Out : Outport
  wires:
  In/1 -> dB Conversion/1
  Input Gain/1 -> Out/1
  dB Conversion/1 -> Input Gain/1

== system commrflib2/Memoryless Nonlinearity/tanh fit/AM_AM ==
  In1 : Inport
  Trigonometric Function : Trigonometry  Operator=tanh
  Out1 : Outport
  wires:
  Trigonometric Function/1 -> Out1/1
  In1/1 -> Trigonometric Function/1

== system commrflib2/Memoryless Nonlinearity/tanh fit/AM_PM ==
  In : Inport
  Input Gain : Gain  Gain=am2pm*pi/180  SaturateOnIntegerOverflow=on
  dB Conversion : dspmathops/dB Conversion  dBtype=dB  intype=Amplitude  R=1  fuzz=on
  Out : Outport
  wires:
  In/1 -> dB Conversion/1
  dB Conversion/1 -> Input Gain/1
  Input Gain/1 -> Out/1

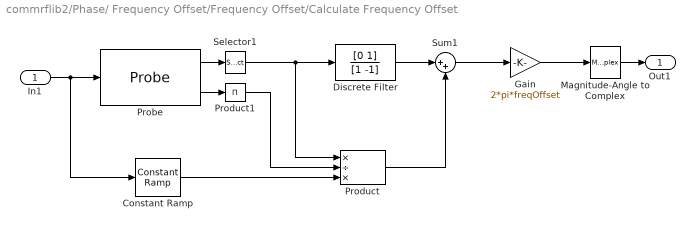
== system commrflib2/Phase/ Frequency Offset/Frequency Offset/Calculate Frequency Offset ==
  In1 : Inport
  Constant Ramp : dspsrcs4/Constant Ramp  L=Rows  Slope=1  Offset=0
  Discrete Filter : DiscreteFilter  Numerator=[0 1]  Denominator=[1 -1]  SampleTime=-1
  Gain : Gain  Gain=2*pi*freqOffset  SaturateOnIntegerOverflow=on
  Magnitude-Angle to Complex : MagnitudeAngleToComplex  Input=Angle  ConstantPart=1
  Probe : Probe  ProbeWidth=off  ProbeComplexSignal=off  ProbeSignalDimensions=on
  Product : Product  Inputs=*/*  SaturateOnIntegerOverflow=on  InputSameDT=on
  Product1 : Product  Inputs=1  SaturateOnIntegerOverflow=on  InputSameDT=on
  Selector1 : Selector  Elements=[1 ]  InputPortWidth=2
  Sum1 : Sum  Inputs=|++  SaturateOnIntegerOverflow=on  InputSameDT=on
  Out1 : Outport
  wires:
  Magnitude-Angle to Complex/1 -> Out1/1
  In1/1 -> Probe/1, Constant Ramp/1
  Probe/2 -> Product1/1
  Product/1 -> Sum1/2
  Probe/1 -> Selector1/1
  Constant Ramp/1 -> Product/3
  Sum1/1 -> Gain/1
  Gain/1 -> Magnitude-Angle to Complex/1
  Product1/1 -> Product/2
  Discrete Filter/1 -> Sum1/1
  Selector1/1 -> Product/1, Discrete Filter/1
